simulink model "uav_trim_sim"  (R2024a)
settings: Solver=VariableStepAuto  StartTime=0.0  StopTime=100  FixedStep=Ts  RelTol=1e-3
values from neighbouring files (symbols this model uses):
  uavParams = make_uav_parameters_eimpc()    [main_sim_eimpc.m]    (also in main_sim_pid.m; make_uav_parameters_eimpc.m = NaN(60,1))
settings Model: Creator=pf  LastModifiedBy=piotr
settings DebuggingCC: InitInArrayFormatMsg=none
settings RTWCC: GPUComputeCapability=3.5

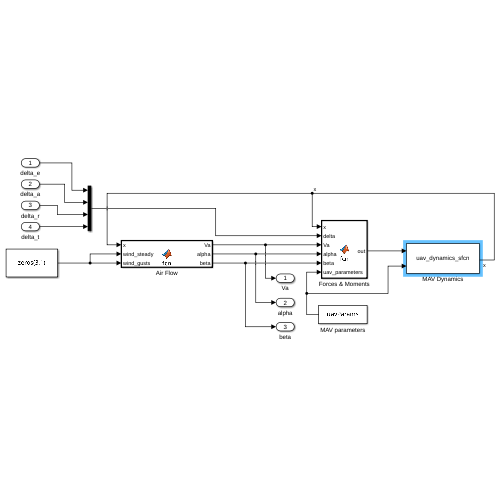
[thumbnail: Simulink's stored preview of the top-level diagram]
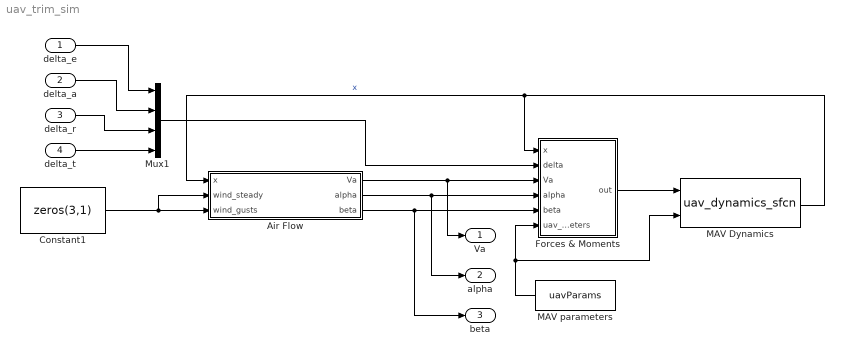
== system uav_trim_sim ==
  delta_e : Inport
  delta_a : Inport  Port=2
  delta_r : Inport  Port=3
  delta_t : Inport  Port=4
  Air Flow : MATLAB Function  TreatAsAtomicUnit=on
  Constant1 : Constant  Value=zeros(3,1)
  Forces & Moments : MATLAB Function  TreatAsAtomicUnit=on
  MAV Dynamics : M-S-Function  FunctionName=uav_dynamics_sfcn  Parameters=x0
  MAV parameters : Constant  Value=uavParams
  Mux1 : Mux
  Va : Outport
  alpha : Outport  Port=2
  beta : Outport  Port=3
  wires:
  Constant1/1 -> Air Flow/3(wind_gusts), Air Flow/2(wind_steady)
  Forces & Moments/1(out) -> MAV Dynamics/1
  Mux1/1 -> Forces & Moments/2(delta)
  Air Flow/3(beta) -> beta/1, Forces & Moments/5(beta)
  delta_e/1 -> Mux1/1
  MAV parameters/1 -> Forces & Moments/6(uav_parameters), MAV Dynamics/2
  Air Flow/2(alpha) -> alpha/1, Forces & Moments/4(alpha)
  delta_r/1 -> Mux1/3
  Air Flow/1(Va) -> Va/1, Forces & Moments/3(Va)
  delta_t/1 -> Mux1/4
  MAV Dynamics/1 -> Air Flow/1(x), Forces & Moments/1(x)  "x"
  delta_a/1 -> Mux1/2

== matlab function uav_trim_sim/Forces & Moments ==
  data: x input; out output; delta input; Va input; alpha input; beta input; uav_parameters input
function out = fcn(x, delta, Va, alpha, beta, uav_parameters)
    out = forces_moments(x, delta, Va, alpha, beta, uav_parameters);
end

== matlab function uav_trim_sim/Air Flow ==
  data: x input; Va output; wind_steady input; wind_gusts input; alpha output; beta output
function [Va, alpha, beta] = fcn(x,wind_steady,wind_gusts)
    [Va, alpha, beta] = airdata(x,wind_steady,wind_gusts);
end
